simulink model "RIEKF"  (R2017b)
settings: Solver=FixedStepDiscrete  StartTime=0.0  StopTime=10  RelTol=1e-3  EnableMultiTasking=on
libraries: lib_StateEstimation x4, dspfdesign x1, slrtlib x1
settings Model: ParamWorkspaceSource=ReferencedWorkspace  Creator=robot  LastModifiedBy=Ross Hartley
settings SolverCC: ConcurrentTasks=on
settings DataIOCC: SaveFormat=Array  SaveOutput=off  SignalLogging=off  DSMLogging=off  VisualizeSimOutput=off  SaveTime=off
settings OptimizationCC: DefaultParameterBehavior=Inlined  InlineInvariantSignals=on  LifeSpan=inf  SimCompilerOptimization=on  AccelVerboseBuild=on
settings DebuggingCC: ReadBeforeWriteMsg=DisableAll  WriteAfterWriteMsg=DisableAll  WriteAfterReadMsg=DisableAll  AllowSymbolicDim=off  SFUnexpectedBacktrackingDiag=warning  SFNoUnconditionalDefaultTransitionDiag=warning  SFExecutionAtInitializationDiag=none
settings HardwareCC: ProdBitPerPointer=32  ProdBitPerSizeT=32  ProdBitPerPtrDiffT=32  ProdLargestAtomicFloat=None  ProdWordSize=32  ProdLongLongMode=on  ProdHWDeviceType=Generic->32-bit x86 compatible
settings ModelReferenceCC: UpdateModelReferenceTargets=IfOutOfDate  ParallelModelReferenceMATLABWorkerInit=Copy Base Workspace  ModelReferenceNumInstancesAllowed=Single
settings SFSimCC: SimUserIncludeDirs=..\..\..\Cassie_Model\gen\kin\src  SFSimEcho=off
settings SFSimCC: SimUserSources=|
  | p_VectorNav_to_RightToeBottom_src.c
  | R_VectorNav_to_RightToeBottom_src.c
  | J_VectorNav_to_RightToeBottom_src.c
  | p_VectorNav_to_LeftToeBottom_src.c
  | R_VectorNav_to_LeftToeBottom_src.c
  | J_VectorNav_to_LeftToeBottom_src.c
settings RTWCC: SystemTargetFile=slrt.tlc  TLCOptions=-axPCMaxOverloads=1000000000 -axPCMaxOverloadLen=1000000000  TemplateMakefile=slrt_default_tmf  Description=Simulink Real-Time  RTWUseSimCustomCode=on  CustomInclude=..\..\..\Cassie_Model\gen\kin\src  CodeExecutionProfiling=on  CodeProfilingSaveOptions=AllData  CodeProfilingInstrumentation=on  RTWCompilerOptimization=on
settings RTWCC: CustomSource=|
  | p_VectorNav_to_RightToeBottom_src.c
  | R_VectorNav_to_RightToeBottom_src.c
  | J_VectorNav_to_RightToeBottom_src.c
  | p_VectorNav_to_LeftToeBottom_src.c
  | R_VectorNav_to_LeftToeBottom_src.c
  | J_VectorNav_to_LeftToeBottom_src.c
settings CodeAppCC: GenerateComments=off  MaxIdLength=128  SimulinkBlockComments=off
settings SimulinkRealTimeCC: ExtMode=off
settings ConfigComp: CovMetricSettings=dw  CovHtmlReporting=on  CovSaveCumulativeToWorkspaceVar=on  CovSaveSingleToWorkspaceVar=on  CovExternalEMLEnable=off

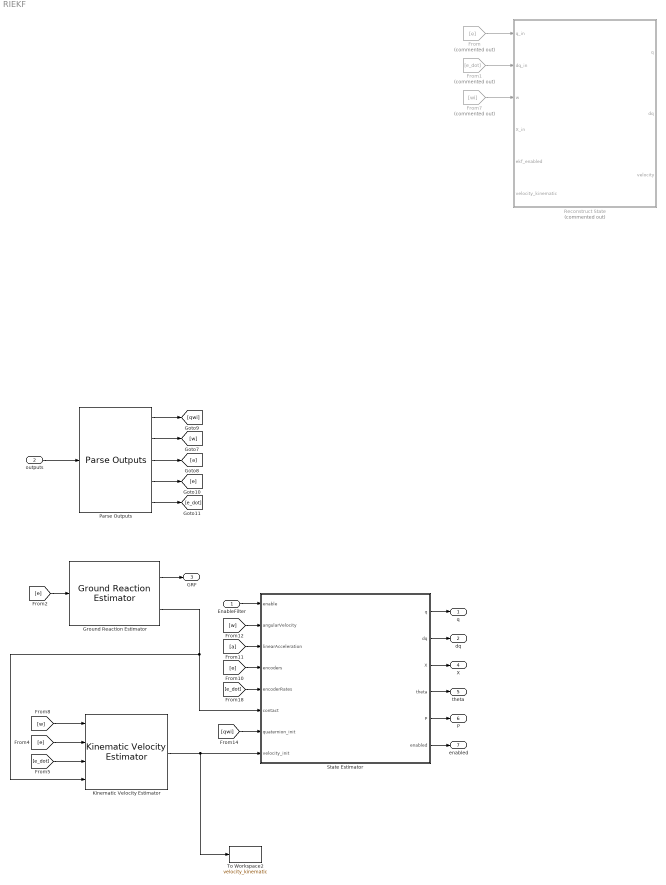
== system RIEKF ==
  EnableFilter : Inport  BusOutputAsStruct=on
  outputs : Inport  Port=2  OutDataTypeStr=Bus: CassieOutBus  BusOutputAsStruct=on
  From : From  Commented=on  GotoTag=e
  From1 : From  Commented=on  GotoTag=e_dot
  From7 : From  Commented=on  GotoTag=wi
  Ground Reaction Estimator : lib_StateEstimation/Ground Reaction Estimator
  Kinematic Velocity Estimator : lib_StateEstimation/Kinematic Velocity Estimator
  Parse Outputs : lib_StateEstimation/Parse Outputs
  Reconstruct State : Subsystem  Commented=on
  State Estimator : Subsystem
  To Workspace2 : ToWorkspace  VariableName=velocity_kinematic  SaveFormat=Timeseries  SampleTime=-1
  q : Outport
  dq : Outport  Port=2
  GRF : Outport  Port=3
  X : Outport  Port=4
  theta : Outport  Port=5
  P : Outport  Port=6
  enabled : Outport  Port=7
  wires:
  Ground Reaction Estimator/2 -> Kinematic Velocity Estimator/4, State Estimator/6(contact)
  [e_dot] -> Kinematic Velocity Estimator/3
  [e] -> Kinematic Velocity Estimator/2
  [w] -> Kinematic Velocity Estimator/1
  Ground Reaction Estimator/1 -> GRF/1
  [e] -> Ground Reaction Estimator/1
  From7/1 -> Reconstruct State/3(w)
  From1/1 -> Reconstruct State/2(dq_in)
  From/1 -> Reconstruct State/1(q_in)
  outputs/1 -> Parse Outputs/1
  Parse Outputs/1 -> [qwi]
  Parse Outputs/2 -> [w]
  Parse Outputs/3 -> [a]
  Parse Outputs/4 -> [e]
  Parse Outputs/5 -> [e_dot]
  EnableFilter/1 -> State Estimator/1(enable)
  [w] -> State Estimator/2(angularVelocity)
  [a] -> State Estimator/3(linearAcceleration)
  [e] -> State Estimator/4(encoders)
  [e_dot] -> State Estimator/5(encoderRates)
  [qwi] -> State Estimator/7(quaternion_init)
  State Estimator/1(q) -> q/1
  State Estimator/2(dq) -> dq/1
  Kinematic Velocity Estimator/1 -> To Workspace2/1, State Estimator/8(velocity_init)
  State Estimator/3(X) -> X/1
  State Estimator/4(theta) -> theta/1
  State Estimator/5(P) -> P/1
  State Estimator/6(enabled) -> enabled/1

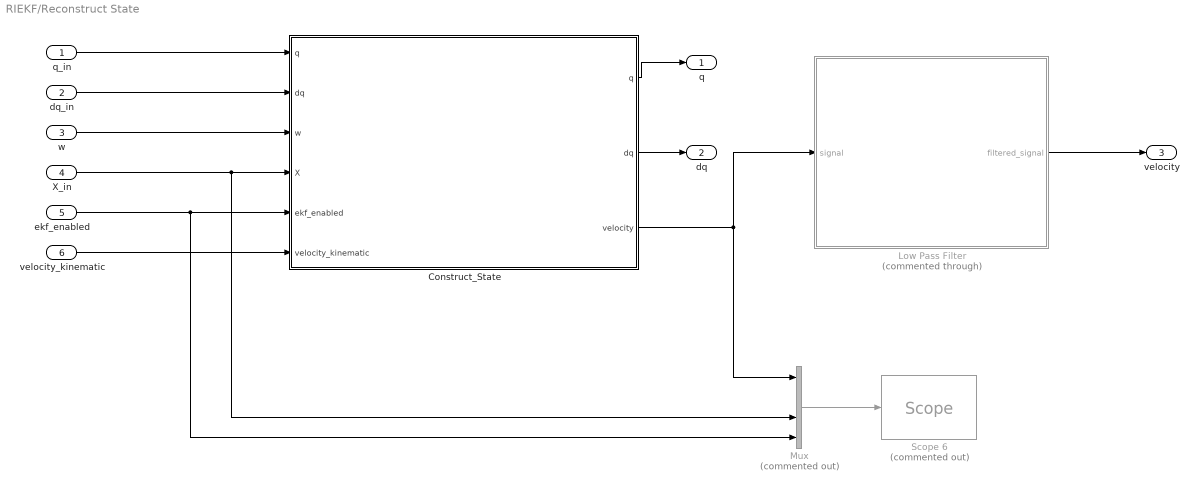
== system RIEKF/Reconstruct State ==
  q_in : Inport
  dq_in : Inport  Port=2
  w : Inport  Port=3
  X_in : Inport  Port=4
  ekf_enabled : Inport  Port=5
  velocity_kinematic : Inport  Port=6
  Construct_State : MATLAB Function  TreatAsAtomicUnit=on
  Low Pass Filter : Subsystem  Commented=through  TreatAsAtomicUnit=on
  Mux : Mux  Commented=on
  Scope 6 : slrtlib/Displays and Logging/Scope   Commented=on  scopeno=6  scopetype=File  autostart=on  viewmode=Numerical  formatstr='%15.6f'  grid=on  ylimits=[0,0]  nosamples=250  noprepostsamples=0  interleave=1  triggermode=FreeRun  triggersignal=1  trigsignalfromport=on  triggerlevel=0.5  triggerslope=Rising  triggerscope=1  triggersample=0  filename=ekf1.dat  mode=Commit  writesize=512  autorestart=on  dynamicfilemode=off  maxwritefilesize=4000*1024^2
  q : Outport
  dq : Outport  Port=2
  velocity : Outport  Port=3
  wires:
  w/1 -> Construct_State/3(w)
  Construct_State/2(dq) -> dq/1
  ekf_enabled/1 -> Mux/4, Construct_State/5(ekf_enabled)
  q_in/1 -> Construct_State/1("q ")
  Mux/1 -> Scope 6/1
  Construct_State/3(velocity) -> Low Pass Filter/1(signal), Mux/1
  Construct_State/1(q) -> q/1
  dq_in/1 -> Construct_State/2("dq ")
  X_in/1 -> Mux/3, Construct_State/4(X)
  Low Pass Filter/1(filtered_signal) -> velocity/1
  velocity_kinematic/1 -> Construct_State/6(velocity_kinematic)

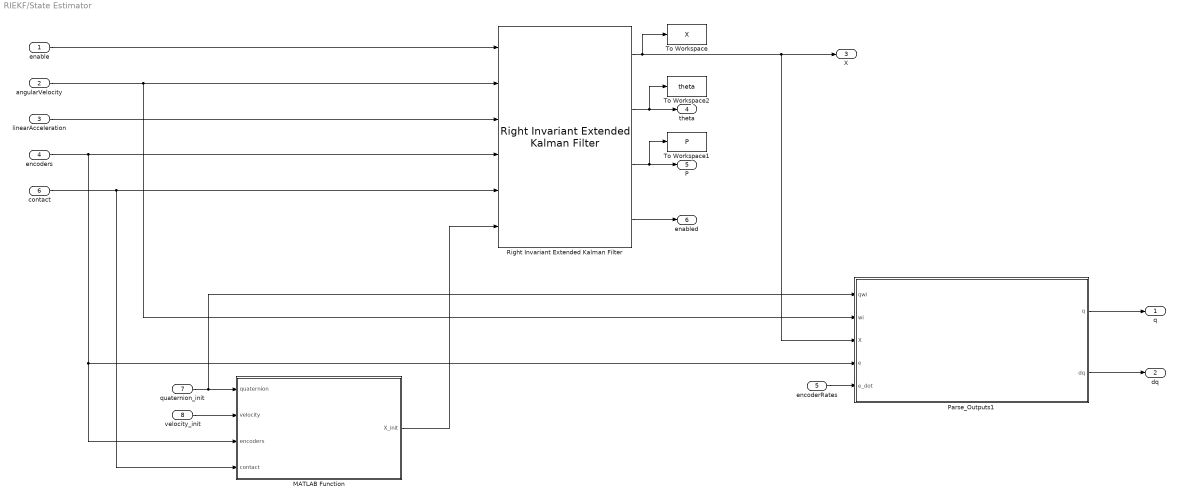
== system RIEKF/State Estimator ==
  enable : Inport
  angularVelocity : Inport  Port=2
  linearAcceleration : Inport  Port=3
  encoders : Inport  Port=4
  encoderRates : Inport  Port=5
  contact : Inport  Port=6
  quaternion_init : Inport  Port=7
  velocity_init : Inport  Port=8
  MATLAB Function : MATLAB Function  TreatAsAtomicUnit=on
  Parse_Outputs1 : MATLAB Function  TreatAsAtomicUnit=on
  Right Invariant Extended Kalman Filter : lib_StateEstimation/Right Invariant Extended Kalman Filter
  To Workspace : ToWorkspace  VariableName=X  SaveFormat=Timeseries  SampleTime=-1
  To Workspace1 : ToWorkspace  VariableName=P  SaveFormat=Timeseries  SampleTime=-1
  To Workspace2 : ToWorkspace  VariableName=theta  SaveFormat=Timeseries  SampleTime=-1
  q : Outport
  dq : Outport  Port=2
  X : Outport  Port=3
  theta : Outport  Port=4
  P : Outport  Port=5
  enabled : Outport  Port=6
  wires:
  enable/1 -> Right Invariant Extended Kalman Filter/1
  angularVelocity/1 -> Right Invariant Extended Kalman Filter/2, Parse_Outputs1/2(wi)
  Right Invariant Extended Kalman Filter/3 -> P/1, To Workspace1/1
  linearAcceleration/1 -> Right Invariant Extended Kalman Filter/3
  velocity_init/1 -> MATLAB Function/2(velocity)
  contact/1 -> Right Invariant Extended Kalman Filter/5, MATLAB Function/4(contact)
  quaternion_init/1 -> Parse_Outputs1/1(qwi), MATLAB Function/1(quaternion)
  MATLAB Function/1(X_init) -> Right Invariant Extended Kalman Filter/6
  encoders/1 -> Right Invariant Extended Kalman Filter/4, Parse_Outputs1/4(e), MATLAB Function/3(encoders)
  Parse_Outputs1/1(q) -> q/1
  encoderRates/1 -> Parse_Outputs1/5(e_dot)
  Right Invariant Extended Kalman Filter/1 -> X/1, Parse_Outputs1/3(X), To Workspace/1
  Parse_Outputs1/2(dq) -> dq/1
  Right Invariant Extended Kalman Filter/2 -> theta/1, To Workspace2/1
  Right Invariant Extended Kalman Filter/4 -> enabled/1

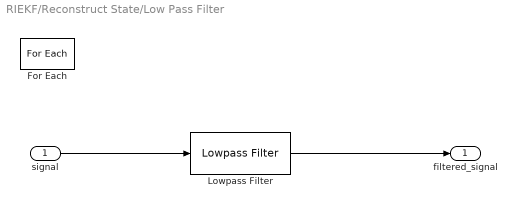
== system RIEKF/Reconstruct State/Low Pass Filter ==
  signal : Inport  Partition=on  PartitionDimension=1  PartitionWidth=1  PartitionOffset=0
  For Each : ForEach  DisableCoverage=on  IndexMode=One-based
  Lowpass Filter : dspfdesign/Lowpass Filter  FilterType=FIR  DesignForMinimumOrder=on  FilterOrder=50  PassbandFrequency=1  StopbandFrequency=10  PassbandRipple=1  StopbandAttenuation=20  InheritSampleRate=off  SampleRate=2000  SimulateUsing=Code generation  roundingMode=Floor  coeffsDataTypeStr=fixdt(1,16)
  filtered_signal : Outport  ConcatenationDimension=1
  wires:
  Lowpass Filter/1 -> filtered_signal/1
  signal/1 -> Lowpass Filter/1

== matlab function RIEKF/State Estimator/Parse_Outputs1 ==
  data: q output; qwi input; wi input; dq output; X input; e input; e_dot input
function [q, dq] = Contruct_State(qwi, wi, X, e, e_dot)   
%   Author: Ross Hartley 
%   Date:   7/03/2017
%

% Compute Euler angles and rates 
Q = Quaternion(qwi);
qq = Q.getEulerAngles();
dqq = Angles.AngularVelocity_to_EulerRates(qq, wi);

% Compute Position and velocity of Pelvis
i_p_ib = [-0.0316; 0; 0.08];
p = X(1:3,5) + X(1:3,1:3)*i_p_ib;
v = X(1:3,4) + X(1:3,1:3)*Angles.skew(wi)*i_p_ib;

% Construct State Vector
q = [p; qq; e];
dq = [v; dqq; e_dot];

end

== matlab function RIEKF/State Estimator/MATLAB Function ==
  data: quaternion input; velocity input; X_init output; encoders input; contact input
function X_init = InitialStateEstimate(quaternion, velocity, encoders, contact)

% R = Angles.Quaternion_to_Rotation(quaternion);
Q = Quaternion(quaternion);
R = Q.getRotation().getValue();
p = zeros(3,1); 
v = R*velocity;
pR = p_VectorNav_to_RightToeBottom(encoders);
pL = p_VectorNav_to_LeftToeBottom(encoders);

if contact(1) == 1
    % Initialize with left foot at 0
    p = -R * pL; % {W}_p_{WL}
elseif contact(2) == 1
    % Initialize with right foot at 0
    p = -R * pR; % {W}_p_{WR}
end

% Initial foot positions
dR = p + R * pR; % {W}_p_{WR}
dL = p + R * pL; % {W}_p_{WL}

% Construct Initial State
X_init = [R, v, p, dR, dL; 0,0,0,1,0,0,0; 0,0,0,0,1,0,0; 0,0,0,0,0,1,0; 0,0,0,0,0,0,1];

% X_init = eye(7);

end

== matlab function RIEKF/Reconstruct State/Construct_State ==
  data: q output; dq output; q input; dq input; w input; X input; ekf_enabled input; velocity output; velocity_kinematic input
function [q, dq, velocity] = Construct_State(q, dq, w, X, ekf_enabled, velocity_kinematic)
% Construct state vector and body velocity estimate using raw data and ekf
%   
%   Inputs:
%       q           - state position vector
%       dq          - state velocity vector
%       w           - angular velocity, {I}_\omega_{WI}
%       contact     - contact indicator
%       X          - EKF state estimate
%       ekf_enabled - EKF enable flag
%
%   Outputs:
%       q                   - 
%       dq                  - 
%       velocity            - EKF body velocity, {W}_v_{WB} 
%       velocity_kinematic  - Kinematic body velocity, {B}_v_{WB} 
%       filter_selector     - used to select low pass filter type
%
%
%   Author: Ross Hartley
%   Date:   11/07/2017

%% Settings
use_ekf_position = true;
use_ekf_orientation = false;
use_ekf_velocity = false;

% Extract encoders
e = q(7:end);

%% Reconstruct State
Rbi = R_VectorNav_to_Pelvis(e)';    % R_{BI}

% Position
if use_ekf_position && ekf_enabled
    Rwi = X(1:3,1:3);
    % {W}_p_{WB} =  {W}_p_{WI} +  {W}_p_{IB}
    q(1:3) = X(1:3,5) + Rwi * p_VectorNav_to_Pelvis(e); 
end

 
% Orientation
if use_ekf_orientation && ekf_enabled
    Rwi = X(1:3,1:3);
    Rwb = Rwi * Rbi';
    q(4:6) = Angles.Rotation_to_Euler( Rwb );
end


% Velocity
if use_ekf_velocity && ekf_enabled
    Rwi = X(1:3,1:3);
    Rwb = Rwi * Rbi';
    % {W}_v_{WB} =  {W}_v_{WI} + R_{WI} * skew({I}_w_{WI}) * {I}_p_{IB}
    dq(1:3) = X(1:3,4) + Rwi * Angles.skew(w) * p_VectorNav_to_Pelvis(e); 
    % {B}_v_{WB} = R_{BW} * {W}_v_{WB}
    velocity = Rwb' * dq(1:3);
else
    Rwb = Angles.Euler_to_Rotation(q(4:6));
    Rwi = Rwb * Rbi;
    % {W}_v_{WB} =  R_{WI} * {I}_v_{WI} + R_{WI} * skew({I}_w_{WI}) * {I}_p_{IB}
    dq(1:3) = Rwi * velocity_kinematic + Rwi * Angles.skew(w) * p_VectorNav_to_Pelvis(e); 
    % {B}_v_{WB} = R_{BW} * {W}_v_{WB}
    velocity = Rwb' * dq(1:3);
end



end
